simulink model "Mdl_13_CloseLoop_w_observer"  (R2018a)
settings: Solver=VariableStepAuto  StartTime=0.0  StopTime=10.0  RelTol=1e-3
undefined symbols (not defined in the file or in its folder): A, B, C, F, G, h, K, L, Ts, x0, x_esht_0
settings Model: Creator=pala  LastModifiedBy=pala
settings DataIOCC: FinalStateName=xF_olwo  SaveFormat=StructureWithTime  SignalLogging=off  DSMLogging=off  StateSaveName=x_olwo  TimeSaveName=t_clwo  OutputSaveName=y_clwo

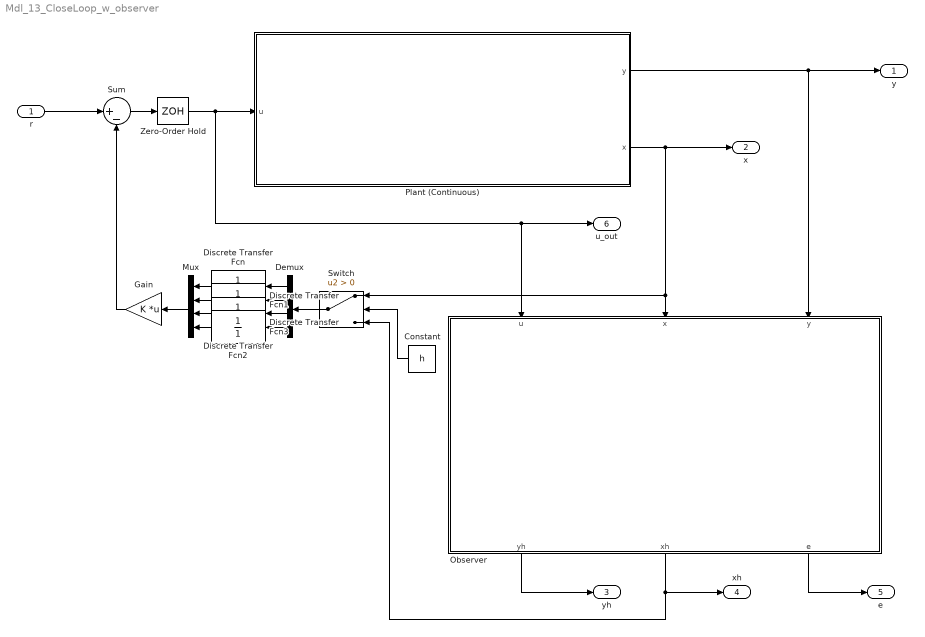
== system Mdl_13_CloseLoop_w_observer ==
  r : Inport  PortDimensions=2
  Constant : Constant  Value=h
  Demux : Demux
  Discrete Transfer Fcn{,1..3} (4 alike) : DiscreteTransferFcn  Denominator=[1]  SampleTime=Ts
  Gain : Gain  Gain=K  Multiplication=Matrix(K*u)
  Mux : Mux
  Observer : Subsystem
  Plant (Continuous) : Subsystem
  Sum : Sum  Inputs=|+-
  Switch : Switch  Criteria=u2 > Threshold
  Zero-Order Hold : ZeroOrderHold  SampleTime=Ts
  y : Outport
  x : Outport  Port=2
  yh : Outport  Port=3
  xh : Outport  Port=4
  e : Outport  Port=5
  u_out : Outport  Port=6
  wires:
  Plant (Continuous)/1(y) -> y/1, Observer/3(y)
  Plant (Continuous)/2(x) -> x/1, Switch/1, Observer/2(x)
  Observer/2(xh) -> Switch/3, xh/1
  Observer/3(e) -> e/1
  Observer/1(yh) -> yh/1
  r/1 -> Sum/1
  Sum/1 -> Zero-Order Hold/1
  Demux/1 -> Discrete Transfer Fcn/1
  Demux/2 -> Discrete Transfer Fcn1/1
  Demux/3 -> Discrete Transfer Fcn2/1
  Demux/4 -> Discrete Transfer Fcn3/1
  Discrete Transfer Fcn/1 -> Mux/1
  Discrete Transfer Fcn1/1 -> Mux/2
  Discrete Transfer Fcn2/1 -> Mux/3
  Discrete Transfer Fcn3/1 -> Mux/4
  Mux/1 -> Gain/1
  Gain/1 -> Sum/2
  Zero-Order Hold/1 -> Observer/1(u), u_out/1, Plant (Continuous)/1(u)
  Switch/1 -> Demux/1
  Constant/1 -> Switch/2

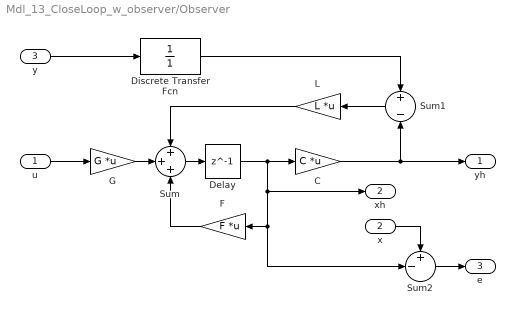
== system Mdl_13_CloseLoop_w_observer/Observer ==
  u : Inport
  x : Inport  Port=2
  y : Inport  Port=3
  C : Gain  Gain=C  Multiplication=Matrix(K*u)
  Delay : Delay  Priority=2  DelayLength=1  InitialCondition=x_esht_0  SampleTime=Ts
  Discrete Transfer Fcn : DiscreteTransferFcn  Denominator=[1]  SampleTime=Ts
  F : Gain  Gain=F  Multiplication=Matrix(K*u)
  G : Gain  Gain=G  Multiplication=Matrix(K*u)
  L : Gain  Gain=L  Multiplication=Matrix(K*u)
  Sum : Sum  Inputs=+++
  Sum1 : Sum  Inputs=+|-
  Sum2 : Sum  Inputs=+-|
  yh : Outport
  xh : Outport  Port=2
  e : Outport  Port=3
  wires:
  G/1 -> Sum/2
  Sum2/1 -> e/1
  y/1 -> Discrete Transfer Fcn/1
  Sum1/1 -> L/1
  Sum/1 -> Delay/1
  F/1 -> Sum/3
  Delay/1 -> C/1, Sum2/2, F/1, xh/1
  u/1 -> G/1
  C/1 -> Sum1/2, yh/1
  L/1 -> Sum/1
  x/1 -> Sum2/1
  Discrete Transfer Fcn/1 -> Sum1/1

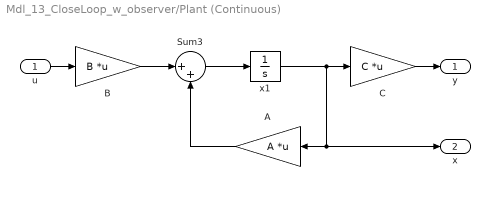
== system Mdl_13_CloseLoop_w_observer/Plant (Continuous) ==
  u : Inport
  A : Gain  Gain=A  Multiplication=Matrix(K*u)
  B : Gain  Gain=B  Multiplication=Matrix(K*u)
  C : Gain  Gain=C  Multiplication=Matrix(K*u)
  Sum3 : Sum  Inputs=|++
  x1 : Integrator  Priority=1  InitialCondition=x0
  y : Outport
  x : Outport  Port=2
  wires:
  A/1 -> Sum3/2
  C/1 -> y/1
  B/1 -> Sum3/1
  u/1 -> B/1
  x1/1 -> C/1, A/1, x/1
  Sum3/1 -> x1/1
